simulink model "testPID_ThreeAxes"  (R2021a)
settings: Solver=VariableStepAuto  StartTime=0.0  StopTime=Torb  RelTol=1e-3
values from neighbouring files (symbols this model uses):
  Tmax = Fmax*Larm    (= 0.00125)    [control_extra2.m]
libraries: simulink x1, sharedtransform x1
settings Model: DataDictionary=databus.sldd  Creator=Laura  LastModifiedBy=Laura

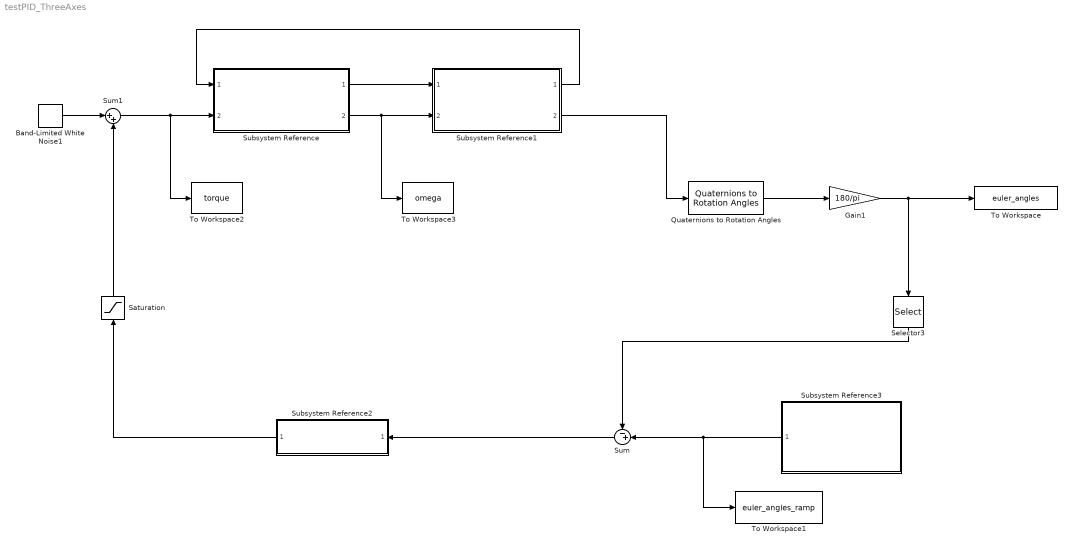
== system testPID_ThreeAxes ==
  Band-Limited White Noise1 : simulink/Sources/Band-Limited White Noise  Cov=[1e-11]  Ts=0.1  seed=[23341]
  Gain1 : Gain  Gain=180/pi
  Quaternions to Rotation Angles : sharedtransform/Quaternions to Rotation Angles  rotationOrder=ZYX  aMode=aMode
      settings: SourceProductBaseCode=AE,PW,DR,MT,UV,VE
  Saturation : Saturate  UpperLimit=Tmax  LowerLimit=-Tmax
  Selector3 : Selector  InputPortWidth=3  IndexOptions=Index vector (dialog)  Indices=[3 2 1]  OutputSizes=1
  Subsystem Reference : Subsystem  ReferencedSubsystem=Dynamics
  Subsystem Reference1 : Subsystem  ReferencedSubsystem=Kinematics
  Subsystem Reference2 : Subsystem  ReferencedSubsystem=PID
  Subsystem Reference3 : Subsystem  ReferencedSubsystem=ThreeAxesSignals
  Sum : Sum  Inputs=-+|
  Sum1 : Sum  Inputs=|++
  To Workspace : ToWorkspace  VariableName=euler_angles  SaveFormat=Timeseries  SampleTime=-1
  To Workspace1 : ToWorkspace  VariableName=euler_angles_ramp  SaveFormat=Timeseries  SampleTime=-1
  To Workspace2 : ToWorkspace  VariableName=torque  SaveFormat=Timeseries  SampleTime=-1
  To Workspace3 : ToWorkspace  VariableName=omega  SaveFormat=Timeseries  SampleTime=-1
  wires:
  Subsystem Reference1/1 -> Subsystem Reference/1
  Subsystem Reference1/2 -> Quaternions to Rotation Angles/1
  Subsystem Reference/2 -> To Workspace3/1, Subsystem Reference1/2
  Subsystem Reference/1 -> Subsystem Reference1/1
  Quaternions to Rotation Angles/1 -> Gain1/1
  Gain1/1 -> Selector3/1, To Workspace/1
  Sum/1 -> Subsystem Reference2/1
  Subsystem Reference2/1 -> Saturation/1
  Band-Limited White Noise1/1 -> Sum1/1
  Selector3/1 -> Sum/1
  Sum1/1 -> To Workspace2/1, Subsystem Reference/2
  Saturation/1 -> Sum1/2
  Subsystem Reference3/1 -> To Workspace1/1, Sum/2
